simulink model "dspstfft"  (Simulink 6.0)
settings: Solver=FixedStepDiscrete  StartTime=0.0  StopTime=0.5  RelTol=1e-3
PreLoadFcn:
  | load mtlb
undefined symbols (not defined in the file or in its folder): jet
libraries: dspbuff3 x2, dspsnks4 x2, dspspect3 x1, dspsrcs4 x1, dspmtrx3 x1, dspmathops x1
settings Model: CovMetricSettings=d  Creator=jeff  LastModifiedBy=mkhan  ProdHWDeviceType=Specified
settings DataIOCC: SaveOutput=off  SaveTime=off  SignalLoggingName=logsOut
settings OptimizationCC: BlockReduction=off  BooleanDataType=off  MultiInstanced=off
settings FormatCC: IgnoreBidirectionalLines=off
settings HardwareCC: ProdHWDeviceType=Specified
settings CodeAppCC: SimulinkBlockComments=off
settings GRTTargetCC: TargetFcnLib=iso_c_tmw.mat

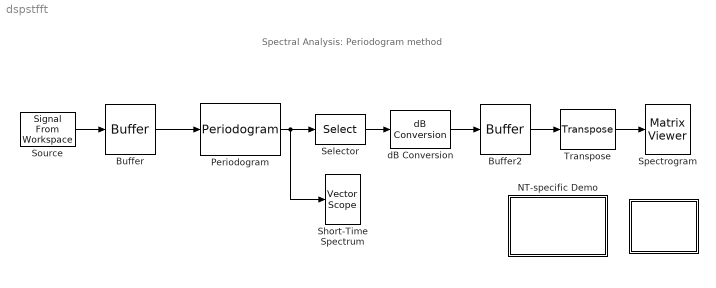
== system dspstfft ==
  note: Spectral Analysis: Periodogram method
  " " : Subsystem
      mask Type: info block for short-time FFT block.
      mask Display: disp('Info')
  Buffer : dspbuff3/Buffer  N=128  V=48  ic=0
  Buffer2 : dspbuff3/Buffer  N=48  V=46  ic=-70
  NT-specific Demo : Subsystem
      settings: OpenFcn=dspstfft_win32
      mask Type: NT-only Demo
      mask Display: disp('PC/Windows\nDemo')
  Periodogram : dspspect3/Periodogram  wintype=Hamming  Rs=50  beta=5  winsamp=Periodic  inheritFFT=on  fftsize=128  navg=2
  Selector : Selector  Elements=1:64  InputPortWidth=128
  Short-Time Spectrum : dspsnks4/Vector Scope  ScopeProperties=on  Domain=Frequency  HorizSpan=1  DisplayProperties=off  AxisGrid=on  Memory=off  FrameNumber=off  AxisLegend=off  AxisZoom=off  OpenScopeAtSimStart=on  OpenScopeImmediately=off  FigPos=[80 110 380 320]  AxisProperties=off  XUnits=Hertz  XRange=[0...Fs/2]  InheritXIncr=on  XIncr=1  XLabel=Samples  YUnits=dB  YLabel=Magnitude, dB  LineProperties=off
      settings: YMin=-59.7576717829863  YMax=9.71199466608513
  Source : dspsrcs4/Signal From Workspace  X=mtlb  Ts=1/8000  nsamps=80  OutputAfterFinalValue=Setting to zero
  Spectrogram : dspsnks4/Matrix Viewer  ImageParams=off  CMapStr=jet(256)  AxisColorbar=on  AxisParams=off  AxisOrigin=Lower left corner  XLabel=Time Index  YLabel=Frequency Index  ZLabel=dB Magnitude  FigPos=[468 110 380 320]  AxisZoom=off
      settings: YMin=-70  YMax=15
  Transpose : dspmtrx3/Transpose  Hermitian=off  overflowFlag=on
  dB Conversion : dspmathops/dB Conversion  dBtype=dB  intype=Amplitude  R=1  fuzz=on
  wires:
  Buffer/1 -> Periodogram/1
  Selector/1 -> dB Conversion/1
  Periodogram/1 -> Short-Time Spectrum/1, Selector/1
  Source/1 -> Buffer/1
  dB Conversion/1 -> Buffer2/1
  Buffer2/1 -> Transpose/1
  Transpose/1 -> Spectrogram/1

== system dspstfft/  ==
  note: Spectral Analysis: Periodogram method
      |
      | This demo illustrates a spectal analysis method known as the periodogram.
      |  Periodogram computes the spectral content of a
      | signal over time, often for the case of a real-time input signal.  The input signal is divided into
      | buffers of equal size, windowed, then an FFT is performed on each buffer of data. The
      | spectrum thus obtained for the short segment of signal is known as the periodogram.

== system dspstfft/NT-specific Demo ==
